simulink model "Experiment4"  (R2023a)
settings: Solver=VariableStepAuto  StartTime=0.0  StopTime=0.01  RelTol=1e-3
libraries: spsDiodeLib x4, spsVoltageMeasurementLib x4, spsACVoltageSourceLib x1, spsSeriesRLCBranchLib x1, spspowerguiLib x1
settings Model: Creator=hp 1  LastModifiedBy=hp 1

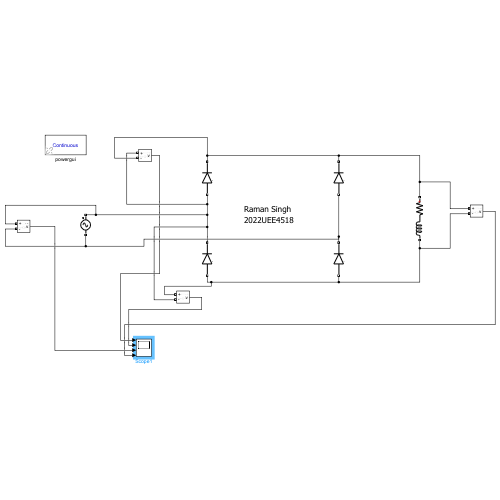
[thumbnail: Simulink's stored preview of the top-level diagram]
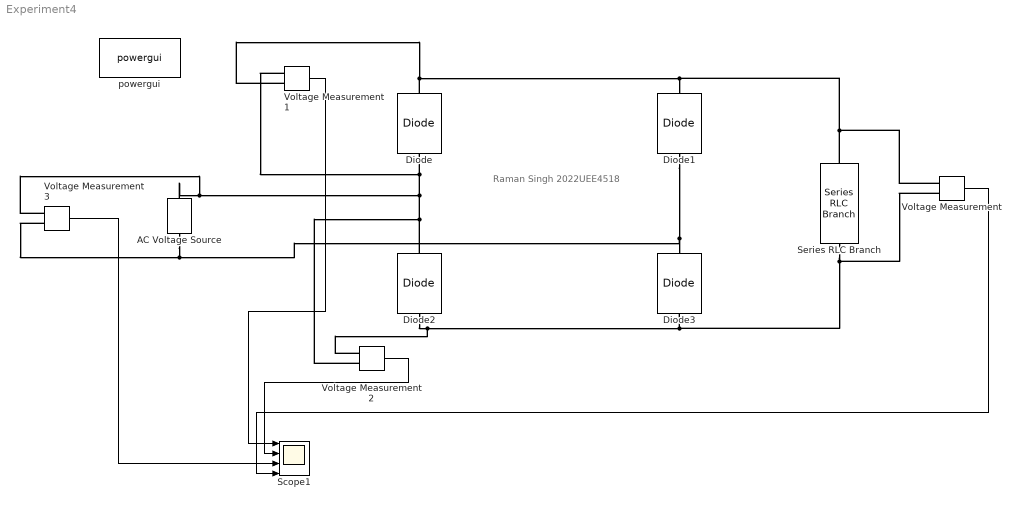
== system Experiment4 ==
  note: Raman Singh
      | 2022UEE4518
  AC Voltage Source : spsACVoltageSourceLib/AC Voltage Source  Amplitude=300  Phase=0  Frequency=100  SampleTime=0  Measurements=None  BusType=swing  Pref=10e3  Qref=0  Qmin=-inf  Qmax=+inf
  Diode{,1..3} (4 alike) : spsDiodeLib/Diode  Ron=0.000001  Lon=0  Vf=0.8  IC=0  UseSnubber=0  Rs=0  Cs=0  Measurements=off
  Scope1 : Scope  NumInputPorts=4
  Series RLC Branch : spsSeriesRLCBranchLib/Series RLC Branch  LConnTagsString=__new0  RConnTagsString=__new0  BranchType=RL  Resistance=100  Inductance=0.001  SetiL0=off  InitialCurrent=0  Capacitance=1e-6  Setx0=off  InitialVoltage=0  Measurements=None
  Voltage Measurement{,1..3} (4 alike) : spsVoltageMeasurementLib/Voltage Measurement  PhasorSimulation=off  OutputType=Complex  PSBequivalent=0
  powergui : spspowerguiLib/powergui  Priority=1  SimulationMode=Continuous  SampleTime=50e-6  frequency=60  Iterations=50  frequencyindice=0  Pbase=100e6  ErrMax=1e-4  UnitsV=kV  UnitsW=MW  buscounter=0  FunctionMessages=off  echomessages=off  EnableUseOfTLC=off  CurrentSourceSwitches=off  DisableSnubberDevices=off  DisableRonSwitches=off  DisableVfSwitches=off  DisplayEquations=off  AutomaticDiscreteSolvers=off  SolverType=Tustin/Backward Euler (TBE)  Interpol=off  ExternalGateDelay=off  methode=off  Ts=100  x0status=blocks  SPID=on  SwTol=0  HookPort=off  NonlinearTolerance=1e-4  nMaxIteration=100  ContinueOnMaxIteration=off  RestoreLinks=warning  ResistiveCurrentMeasurement=off  Frange=[0:2:500]  Ylog=off  Xlog=on  ShowGrid=off  save=off  variable=ZData  structure=0  ZoomFFT=off  StartTime=0.0  cycles=1  DisplayStyle=1  fundamental=60  FreqAxis=off  MaxFrequency=1000  frequencyindicesteady=1  RmsSteady=1  display=off
  wires:
  Voltage Measurement3/1 -> Scope1/3
  Voltage Measurement1/1 -> Scope1/1
  Voltage Measurement2/1 -> Scope1/2
  Voltage Measurement/1 -> Scope1/4
  connections:
  Diode2/RConn1 -- Voltage Measurement3/LConn1 -- AC Voltage Source/RConn1 -- Voltage Measurement1/LConn1 -- Diode/LConn1 -- Voltage Measurement2/LConn2
  Diode/RConn1 -- Voltage Measurement1/LConn2 -- Voltage Measurement/LConn1 -- Series RLC Branch/LConn1 -- Diode1/RConn1
  Diode2/LConn1 -- Voltage Measurement2/LConn1 -- Voltage Measurement/LConn2 -- Series RLC Branch/RConn1 -- Diode3/LConn1
  AC Voltage Source/LConn1 -- Diode1/LConn1 -- Diode3/RConn1 -- Voltage Measurement3/LConn2
